simulink model "verify_Inverter_SPI_mdl"  (R2018b)
settings: Solver=FixedStepAuto  StartTime=tsim_start  StopTime=tsim_end  FixedStep=Tstest  RelTol=1e-3
values from neighbouring files (symbols this model uses):
  useAcCharge = 0    [InputData_verify.mat]
undefined symbols (not defined in the file or in its folder): path_carnot, phase
libraries: carnot x3
settings Model: SimulationMode=accelerator  PauseTimes=54194  Creator=P41573  LastModifiedBy=drhf
settings DataIOCC: SaveFormat=Array  SignalLogging=off  DSMLogging=off  ReturnWorkspaceOutputsName=simout
settings OptimizationCC: EfficientMapNaN2IntZero=off
settings HardwareCC: TargetBitPerPointer=64  TargetBitPerSizeT=64  TargetBitPerPtrDiffT=64  TargetLongLongMode=on  TargetIntDivRoundTo=Zero  TargetEndianess=LittleEndian  TargetWordSize=64  TargetHWDeviceType=MATLAB Host  ProdEqTarget=off
settings CodeAppCC: MaxIdLength=128
settings GRTTargetCC: TargetLangStandard=C89/C90 (ANSI)  CombineOutputUpdateFcns=off  GRTInterface=on

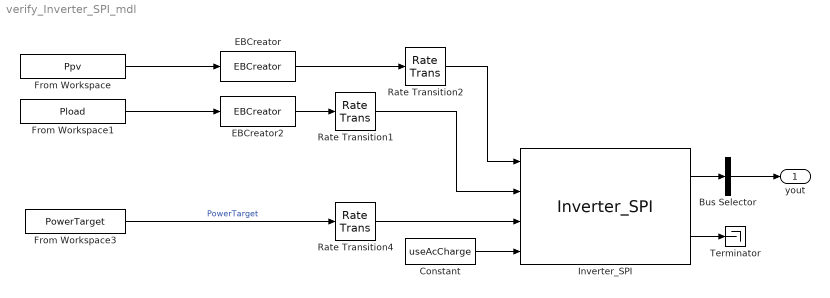
== system verify_Inverter_SPI_mdl ==
  Bus Selector : BusSelector  OutputSignals=Ppvbs,Ppv2ac,Pbat2ac,Ppv2bat,SOC,Ppv,Pload  OutputAsBus=on
  Constant : Constant  Value=useAcCharge
  EBCreator : carnot/Basic/Electric/EBCreator  Inport_ID=off  Inport_f=off  Inport_v1=off  Inport_p1=on  Inport_pf1=off  Inport_v2=off  Inport_p2=off  Inport_pf2=off  Inport_v3=off  Inport_p3=off  Inport_pf3=off  ID=1  f=0  v1=0  p1=1e5  pf1=1  v2=0  p2=0  pf2=0  v3=0  p3=0  pf3=0  Annotation_ID=off  Annotation_f=off  Annotation_v1=off  Annotation_p1=off  Annotation_pf1=off  Annotation_v2=off  Annotation_p2=off  Annotation_pf2=off  Annotation_v3=off  Annotation_p3=off  Annotation_pf3=off
      settings: SourceProductName=Carnot
  EBCreator2 : carnot/Basic/Electric/EBCreator  Inport_ID=off  Inport_f=off  Inport_v1=off  Inport_p1=on  Inport_pf1=off  Inport_v2=off  Inport_p2=off  Inport_pf2=off  Inport_v3=off  Inport_p3=off  Inport_pf3=off  ID=1  f=50  v1=240  p1=1e5  pf1=1  v2=0  p2=0  pf2=0  v3=0  p3=0  pf3=0  Annotation_ID=on  Annotation_f=on  Annotation_v1=on  Annotation_p1=off  Annotation_pf1=off  Annotation_v2=off  Annotation_p2=off  Annotation_pf2=off  Annotation_v3=off  Annotation_p3=off  Annotation_pf3=off
      settings: SourceProductName=Carnot
      settings: AttributesFormatString=|
      | ID 1
      | 50 Hz frequency
      | 240 V Voltage
  From Workspace : FromWorkspace  VariableName=Ppv  SampleTime=1  Interpolate=off  OutputAfterFinalValue=Setting to zero
  From Workspace1 : FromWorkspace  VariableName=Pload  SampleTime=1  Interpolate=off  OutputAfterFinalValue=Setting to zero
  From Workspace3 : FromWorkspace  VariableName=PowerTarget  SampleTime=1  Interpolate=off  OutputAfterFinalValue=Setting to zero
  Inverter_SPI : carnot/Source/Electric_Generator/Inverter_SPI  PathName=fullfile(path_carnot('libsl'), 'Source', 'Electric_Generator', 'Inverter_SPI', 'parameter_set')  FileName='InverterSPI_Default_5p5kW_11p5kWh.mat'  userPath=off  userParam=off  nphase=3-phase  soc0=0.2  socMin=0  socMax=1  Tsample=1  capUser=0  SpiData=[5.686;5.487;6.35626283367556;6.191;5.419;0;73.4437227313543;94.5955883042527;31.1212070123701;74.9053455860837;92.4754002317794;31.7469866284786;30.8769273130404;90.5542640263268;41.6993897221684;86.4449570278825;105.13781756438;31.4770198650726;1;1;1;1;1;1;0.98;0.98;1.32333333333333;0.15;0;4.47;4.56;1.55;10.7670579897002;95.2833]
      settings: SourceProductName=Carnot
  Rate Transition1 : RateTransition  Integrity=off  OutPortSampleTime=Tstest
  Rate Transition2 : RateTransition  Integrity=off  OutPortSampleTime=Tstest
  Rate Transition4 : RateTransition  Integrity=off  OutPortSampleTime=Tstest
  Terminator : Terminator
  yout : Outport
  wires:
  From Workspace3/1 -> Rate Transition4/1  "PowerTarget"
  From Workspace1/1 -> EBCreator2/1
  From Workspace/1 -> EBCreator/1
  EBCreator/1 -> Rate Transition2/1
  Constant/1 -> Inverter_SPI/4
  Inverter_SPI/1 -> Bus Selector/1
  EBCreator2/1 -> Rate Transition1/1
  Rate Transition2/1 -> Inverter_SPI/1
  Rate Transition1/1 -> Inverter_SPI/2
  Inverter_SPI/2 -> Terminator/1
  Bus Selector/1 -> yout/1
  Rate Transition4/1 -> Inverter_SPI/3
